simulink model "test_newfft_4"  (Simulink 7.0)
settings: Solver=ode45  StartTime=0.0  StopTime=100  RelTol=1e-3
libraries: xbsIndex_r4 x135, simulink x1, casper_library x1
(part 1 of 3)
settings Model: Creator=homin  LastModifiedBy=homin
settings DebuggingCC: SaveWithParameterizedLinksMsg=none  SignalResolutionControl=TryResolveAllWithWarning  MultiTaskDSMMsg=warning  MultiTaskCondExecSysMsg=none  StrictBusMsg=None
settings RTWCC: IncludeERTFirstTime=on
settings GRTTargetCC: TargetFcnLib=ansi_tfl_tmw.mat

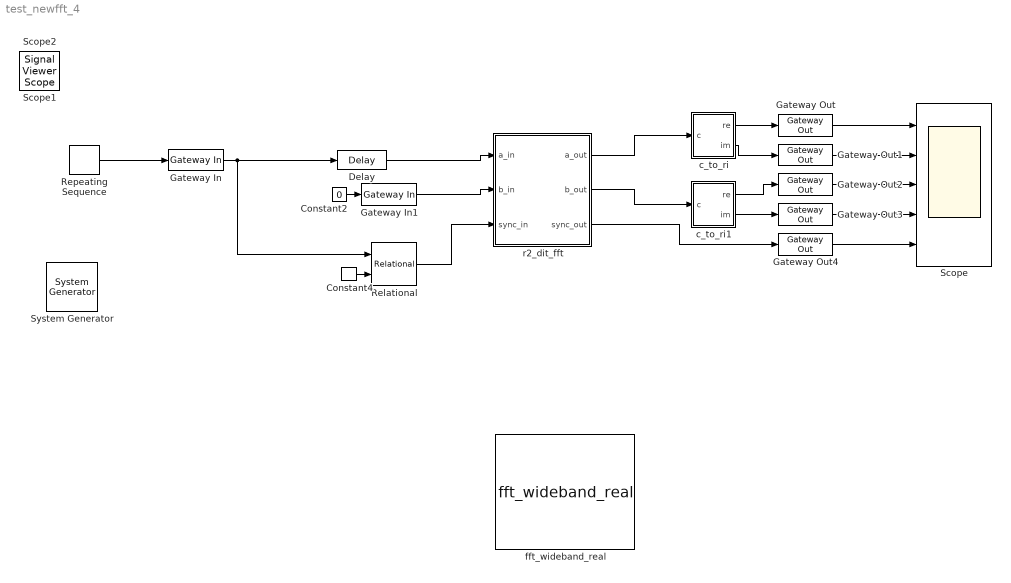
== system test_newfft_4 ==
  " System Generator" : xbsIndex_r4/ System Generator  Tag=genX  SystemSampleTime=-1  xilinxfamily=Virtex2  part=xc2v1000  speed=-4  package=bg575  synthesis_tool=XST  clock_wrapper=Clock Enables  directory=./netlist  testbench=off  simulink_period=1  sysclk_period=100  dcm_input_clock_period=100  incr_netlist=off  trim_vbits=Everywhere in SubSystem  dbl_ovrd=According to Block Masks  core_generation=According to Block Masks  run_coregen=off  deprecated_control=off  eval_field=0  block_type=sysgen
      settings: block_version=10.1.3
  Constant2 : Constant  Value=0  OutDataType=sfix(16)  OutScaling=2^0
  Constant4 : xbsIndex_r4/Constant  arith_type=Unsigned  const=0  n_bits=16  bin_pt=0  explicit_period=off  period=1  equ=P=C  opselect=C  inp2=PCIN>>17  opr=+  inp1=P  carry=CIN  dbl_ovrd=off  block_type=constant
  Delay : xbsIndex_r4/Delay  en=off  latency=2  dbl_ovrd=off  reg_retiming=off  block_type=delay
      settings: xl_area=[0, 0, 0, 0, 0, 0, 0]
  Gateway In : xbsIndex_r4/Gateway In  arith_type=Unsigned  n_bits=16  bin_pt=0  quantization=Truncate  overflow=Wrap  period=1  dbl_ovrd=off  timing_constraint=None  locs_specified=off  LOCs={}  block_type=gatewayin
      settings: infoedit="Gateway in block.  Converts inputs of type Simulink integer, double and fixed point to  Xilinx fixed point type.<P><P>Hardware notes:  In hardware these blocks become top level input ports."  xl_area=[0, 0, 0, 0, 0, 0, 0]  block_version=10.1.3
  Gateway In1 : xbsIndex_r4/Gateway In  arith_type=Unsigned  n_bits=16  bin_pt=0  quantization=Truncate  overflow=Wrap  period=1  dbl_ovrd=off  timing_constraint=None  locs_specified=off  LOCs={}  block_type=gatewayin
      settings: infoedit="Gateway in block.  Converts inputs of type Simulink integer, double and fixed point to  Xilinx fixed point type.<P><P>Hardware notes:  In hardware these blocks become top level input ports."  xl_area=[0, 0, 0, 0, 0, 0, 0]  block_version=10.1.3
  Gateway Out{,1..4} (5 alike) : xbsIndex_r4/Gateway Out  hdl_port=on  timing_constraint=None  locs_specified=off  LOCs={}  block_type=gatewayout
      settings: infoedit="Gateway out block.  Converts Xilinx fixed point inputs into ouputs of type Simulink integer, double, or fixed point.<P><P>Hardware notes:  In hardware these blocks become top level output ports or are discarded, depending on how they are configured."  xl_area=[0, 0, 0, 0, 0, 0, 0]  block_version=10.1.3
  Relational : xbsIndex_r4/Relational  mode=a!=b  en=off  latency=0  dbl_ovrd=off  block_type=relational
      settings: xl_area=[0, 0, 0, 0, 0, 0, 0]  block_version=10.1.3
  Repeating Sequence : simulink/Sources/Repeating Sequence  SystemSampleTime=-1  rep_seq_t=[0:16]  rep_seq_y=[1 zeros(1,15) 1]*hex2dec('7f00')
  Scope : Scope  NumInputPorts=5
      settings: YMin=-5~-5~-5~-5~-5  YMax=5~5~5~5~5
  c_to_ri : Subsystem  mask(Complex to Real-Imag){n_bits=10, bin_pt=7}
      mask prompts: n_bits "Bit Width"; bin_pt "Binary Point"
      mask help: Outputs real and imaginary components of a complex input.
      mask init:
      | c_to_ri_init(gcb,n_bits,bin_pt);
      settings: AttributesFormatString=10_7 r/i
      mask Help:
      | <pre>
      | Description::
      | 
      | Outputs real and imaginary components of a complex input.
      | Useful for simplifying interconnects.
      | See also: Real-Imag to Complex (ri_to_c)
      | 
      | Mask Parameters::
      | 
      | Bit Width (n_bits): Specifies the width of the real/imaginary components.
      | Assumed equal for both components.
      | 
      | Binary Point (bin_pt): Specifies the binary point location in the real/imaginary components.
      | Assumed equal for both components.
      | </pre>
  c_to_ri1 : Subsystem  mask(Complex to Real-Imag){n_bits=10, bin_pt=7}
      mask prompts: n_bits "Bit Width"; bin_pt "Binary Point"
      mask help: Outputs real and imaginary components of a complex input.
      mask init:
      | c_to_ri_init(gcb,n_bits,bin_pt);
      settings: AttributesFormatString=10_7 r/i
      mask Help:
      | <pre>
      | Description::
      | 
      | Outputs real and imaginary components of a complex input.
      | Useful for simplifying interconnects.
      | See also: Real-Imag to Complex (ri_to_c)
      | 
      | Mask Parameters::
      | 
      | Bit Width (n_bits): Specifies the width of the real/imaginary components.
      | Assumed equal for both components.
      | 
      | Binary Point (bin_pt): Specifies the binary point location in the real/imaginary components.
      | Assumed equal for both components.
      | </pre>
  fft_wideband_real : casper_library/FFTs/fft_wideband_real  SystemSampleTime=-1  FFTSize=5  input_bit_width=18  coeff_bit_width=18  n_inputs=2  quantization=Truncate  overflow=Wrap  add_latency=2  mult_latency=3  bram_latency=2  arch=Virtex2Pro  opt_target=Multipliers  coeffs_bit_limit=8  delays_bit_limit=9  specify_mult=off  mult_spec=[2 2 2 2 2]  dsp48_adders=off
      link override fft_direct/butterfly1_0/convert_of1/all_0s: logical_function=NAND  inputs=5  latency=latency  precision=Full
      link override fft_direct/butterfly1_0/convert_of1/all_1s: logical_function=NAND  inputs=5  latency=latency  precision=Full
      link override fft_direct/butterfly1_0/convert_of1/and: logical_function=AND  inputs=2  latency=0  precision=Full
      link override fft_direct/butterfly1_0/convert_of1/convert: n_bits=bit_width_o  bin_pt=binary_point_o  quantization=Truncate  overflow=Wrap  latency=latency  pipeline=on
      link override fft_direct/butterfly1_0/convert_of1/din: Port=1
      link override fft_direct/butterfly1_0/convert_of1/dout: Port=1
      link override fft_direct/butterfly1_0/convert_of1/of: Port=2
      link override fft_direct/butterfly1_0/convert_of1/slice1: boolean_output=on  mode=Upper Bit Location + Width  bit1=0  base1=MSB of Input
      link override fft_direct/butterfly1_0/convert_of1/slice2: boolean_output=on  mode=Upper Bit Location + Width  bit1=-1  base1=MSB of Input
      link override fft_direct/butterfly1_0/convert_of1/slice3: boolean_output=on  mode=Upper Bit Location + Width  bit1=-2  base1=MSB of Input
      link override fft_direct/butterfly1_0/convert_of1/slice4: boolean_output=on  mode=Upper Bit Location + Width  bit1=-3  base1=MSB of Input
      link override fft_direct/butterfly1_0/convert_of1/slice5: boolean_output=on  mode=Upper Bit Location + Width  bit1=-4  base1=MSB of Input
      link override fft_direct/butterfly1_0/convert_of2/all_0s: logical_function=NAND  inputs=5  latency=latency  precision=Full
      link override fft_direct/butterfly1_0/convert_of2/all_1s: logical_function=NAND  inputs=5  latency=latency  precision=Full
      link override fft_direct/butterfly1_0/convert_of2/and: logical_function=AND  inputs=2  latency=0  precision=Full
      link override fft_direct/butterfly1_0/convert_of2/convert: n_bits=bit_width_o  bin_pt=binary_point_o  quantization=Truncate  overflow=Wrap  latency=latency  pipeline=on
      link override fft_direct/butterfly1_0/convert_of2/din: Port=1
      link override fft_direct/butterfly1_0/convert_of2/dout: Port=1
      link override fft_direct/butterfly1_0/convert_of2/of: Port=2
      link override fft_direct/butterfly1_0/convert_of2/slice1: boolean_output=on  mode=Upper Bit Location + Width  bit1=0  base1=MSB of Input
      link override fft_direct/butterfly1_0/convert_of2/slice2: boolean_output=on  mode=Upper Bit Location + Width  bit1=-1  base1=MSB of Input
      link override fft_direct/butterfly1_0/convert_of2/slice3: boolean_output=on  mode=Upper Bit Location + Width  bit1=-2  base1=MSB of Input
      link override fft_direct/butterfly1_0/convert_of2/slice4: boolean_output=on  mode=Upper Bit Location + Width  bit1=-3  base1=MSB of Input
      link override fft_direct/butterfly1_0/convert_of2/slice5: boolean_output=on  mode=Upper Bit Location + Width  bit1=-4  base1=MSB of Input
      link override fft_direct/butterfly1_0/convert_of3/all_0s: logical_function=NAND  inputs=5  latency=latency  precision=Full
      link override fft_direct/butterfly1_0/convert_of3/all_1s: logical_function=NAND  inputs=5  latency=latency  precision=Full
      link override fft_direct/butterfly1_0/convert_of3/and: logical_function=AND  inputs=2  latency=0  precision=Full
      link override fft_direct/butterfly1_0/convert_of3/convert: n_bits=bit_width_o  bin_pt=binary_point_o  quantization=Truncate  overflow=Wrap  latency=latency  pipeline=on
      link override fft_direct/butterfly1_0/convert_of3/din: Port=1
      link override fft_direct/butterfly1_0/convert_of3/dout: Port=1
      link override fft_direct/butterfly1_0/convert_of3/of: Port=2
      link override fft_direct/butterfly1_0/convert_of3/slice1: boolean_output=on  mode=Upper Bit Location + Width  bit1=0  base1=MSB of Input
      link override fft_direct/butterfly1_0/convert_of3/slice2: boolean_output=on  mode=Upper Bit Location + Width  bit1=-1  base1=MSB of Input
      link override fft_direct/butterfly1_0/convert_of3/slice3: boolean_output=on  mode=Upper Bit Location + Width  bit1=-2  base1=MSB of Input
      link override fft_direct/butterfly1_0/convert_of3/slice4: boolean_output=on  mode=Upper Bit Location + Width  bit1=-3  base1=MSB of Input
      link override fft_direct/butterfly1_0/convert_of3/slice5: boolean_output=on  mode=Upper Bit Location + Width  bit1=-4  base1=MSB of Input
      link override fft_direct/butterfly1_0/convert_of4/all_0s: logical_function=NAND  inputs=5  latency=latency  precision=Full
      link override fft_direct/butterfly1_0/convert_of4/all_1s: logical_function=NAND  inputs=5  latency=latency  precision=Full
      link override fft_direct/butterfly1_0/convert_of4/and: logical_function=AND  inputs=2  latency=0  precision=Full
      link override fft_direct/butterfly1_0/convert_of4/convert: n_bits=bit_width_o  bin_pt=binary_point_o  quantization=Truncate  overflow=Wrap  latency=latency  pipeline=on
      link override fft_direct/butterfly1_0/convert_of4/din: Port=1
      link override fft_direct/butterfly1_0/convert_of4/dout: Port=1
      link override fft_direct/butterfly1_0/convert_of4/of: Port=2
      link override fft_direct/butterfly1_0/convert_of4/slice1: boolean_output=on  mode=Upper Bit Location + Width  bit1=0  base1=MSB of Input
      link override fft_direct/butterfly1_0/convert_of4/slice2: boolean_output=on  mode=Upper Bit Location + Width  bit1=-1  base1=MSB of Input
      link override fft_direct/butterfly1_0/convert_of4/slice3: boolean_output=on  mode=Upper Bit Location + Width  bit1=-2  base1=MSB of Input
      link override fft_direct/butterfly1_0/convert_of4/slice4: boolean_output=on  mode=Upper Bit Location + Width  bit1=-3  base1=MSB of Input
      link override fft_direct/butterfly1_0/convert_of4/slice5: boolean_output=on  mode=Upper Bit Location + Width  bit1=-4  base1=MSB of Input
      link override fft_direct/butterfly1_0/twiddle/convert_of/convert: n_bits=bit_width_o  bin_pt=binary_point_o  quantization=Truncate  overflow=Wrap  latency=latency  pipeline=on
      link override fft_direct/butterfly1_0/twiddle/convert_of/din: Port=1
      link override fft_direct/butterfly1_0/twiddle/convert_of/dout: Port=1
      link override fft_direct/butterfly1_0/twiddle/convert_of/never: arith_type=Boolean  const=0  explicit_period=on  period=1
      link override fft_direct/butterfly1_0/twiddle/convert_of/of: Port=2
      link override fft_direct/butterfly1_0/twiddle/convert_of1/convert: n_bits=bit_width_o  bin_pt=binary_point_o  quantization=Truncate  overflow=Wrap  latency=latency  pipeline=on
      link override fft_direct/butterfly1_0/twiddle/convert_of1/din: Port=1
      link override fft_direct/butterfly1_0/twiddle/convert_of1/dout: Port=1
      link override fft_direct/butterfly1_0/twiddle/convert_of1/never: arith_type=Boolean  const=0  explicit_period=on  period=1
      link override fft_direct/butterfly1_0/twiddle/convert_of1/of: Port=2
      link override fft_direct/butterfly1_0/twiddle/convert_of2/convert: n_bits=bit_width_o  bin_pt=binary_point_o  quantization=Truncate  overflow=Wrap  latency=latency  pipeline=on
      link override fft_direct/butterfly1_0/twiddle/convert_of2/din: Port=1
      link override fft_direct/butterfly1_0/twiddle/convert_of2/dout: Port=1
      link override fft_direct/butterfly1_0/twiddle/convert_of2/never: arith_type=Boolean  const=0  explicit_period=on  period=1
      link override fft_direct/butterfly1_0/twiddle/convert_of2/of: Port=2
      settings: AttributesFormatString=FFTSize=5
  r2_dit_fft : Subsystem  AncestorBlock=newfft_library/FFT/r2_dit_fft  mask(Biplex Radix-2 DIT FFT){n_stages=2, n_bits=8, bin_pt=7, shifts=[0], commutator_bram=0, twiddle_bram=0, n_bits_w=9, mult_latency=3, add_latency=1, commute_output=Yes (SLR16), output_order=Normal, show_sbo=on, munge_submasks=DumbDown}
      mask prompts: n_stages "Total Stages"; n_bits "Number of Bits In"; bin_pt "Binary Point In"; shifts "Shifting Schedule"; commutator_bram "Number of Stages Using BRAM for Biplex Commutators (i.e. delays)"; twiddle_bram "Number of Stages Using BRAM for Twiddle Coefficients"; n_bits_w "Twiddle Coefficient Bitwidth"; mult_latency "Multiplier Latency"; add_latency "Adder Latency"; commute_output "Commute Output"; output_order "Output Order"; show_sbo "Show Sub-Block Options"; munge_submasks "Sub-Block Masks"
      mask help: A biplex radix-2 decimation-in-time Fast Fourier Transform.
      mask init:
      | tic
      | r2_dit_fft_init(gcb, ...
      |   n_stages, ...
      |   n_bits, ...
      |   bin_pt, ...
      |   shifts, ...
      |   commutator_bram, ...
      |   twiddle_bram, ...
      |   n_bits_w, ...
      |   mult_latency, ...
      |   add_latency, ...
      |   commute_output, ...
      |   output_order, ...
      |   lower(get_param(gcb,'munge_submasks')) );
      | disp('r2_dit_fft initialization complete.');
      | toc
      settings: AttributesFormatString=|
      | 4 points
      | 8_7 r/i in
      | 9_7 twiddles
      mask Help:
      | <pre>
      | Description::
      | 
      | A biplex radix-2 decimation-in-time Fast Fourier Transform.
      | 
      | The two inputs to the biplex FFT are independent complex signals (e.g. A and B).
      | 
      | Without an output commutator, the two outputs of the FFT are commuted such that the a_out
      | signal is really the "lower" half of A's transform followed by the "lower" half of B's
      | transform and b_out is really the "upper" half of A's transform followed by the "upper"
      | half of B's transform.
      | 
      | If it is desired to have the two halves of A's transform follow each other on the same path
      | and the two halves of B's transform follow each other on the same path, then be sure to
      | check the "Output Commutator" checkbox.  This will result in the "lower" half of A (or B)
      | followed by the "upper" half of A (or B).  Including the output commutator uses additional
      | resources.
      | 
      | If the "Normal" Ouput Order option is chosen, the output will be in normal order (though still in
      | commuted halves if no output commutator is used).  If the "Bit Reversed" Output Order" option is
      | selected, the output halves (either commuted or not) will each be in bit reversed order
      | (i.e. each half of each transform will be in bit reversed output order).   Normal output is easier
      | for humans to work with (especially for testing), but it uses additional resources.  Bit reversed
      | output is the implementation's inhernet output order so that option uses no additional resources.
      | 
      | The number of bits for each real and imaginary component grows by two through each stage.
      | If a stage's input bit width is 17 or less, three embedded multipliers will be used per complex multiply.
      | If a stage's input bit width is 18, four embedded multipliers will be used per complex multiply.
      | If a stage's input bit width exceeds 18, then substantially more embedded multipliers will be used
      | per complex multiply.  Enabling "shifting" in some (or all) stages can limit the bit growth
      | to prevent this.  See the Shifting Schedule parameter for more info.
      | 
      | Mask Parameters::
      | 
      | Total Stages (n_stages):  The number of total stages in the FFT.
      | The FFT will have 2^n_stages points.
      | 
      | Number of Bits In (n_bits): Specifies the width of the real/imaginary components of ports
      | a_in and b_in.  Assumed equal for both components.  The output bit width will be
      | n_bits+n_stages (assuming sum(shifts)==0).
      | 
      | Binary Point In (bin_pt): Specifies the binary point position of the real/imaginary
      | components of ports a_in and b_in.  Assumed equal for both components.
      | 
      | Shifting Schedule (shifts): A vector specifying how many bits to shift by at each stage.
      | Missing values are assumed to be zero; extra values are ignored.
      | 
      | Number of Stages Using BRAM for Biplex Commutators (commutator_bram): Number of stages
      | that will use BRAM for commutator memory.  Remaining stages will use SLR16 elements (slices).
      | 
      | Number of Stages Using BRAM for Twiddle Coefficients (twiddle_bram): Number of stages that
      | will use BRAM for twiddle coeeficient storage.  Remaining stages will use distributed memory
      | (slices).
      | 
      | Twiddle Coefficient Bitwidth (n_bits_w): Specifies the width of the real/imaginary
      | components of the twiddle coefficients.  Assumed equal for both components.
      | 
      | Multiplier Latency (mult_latency): Latency to use for the underlying real multipliers.
      | 
      | Adder Latency (add_latency): Latency to use for the underlying real adders.
      | 
      | Commute Output (commute_output): Popup options for an output commutator.  See decription
      | above for details on the output commutator.  Choices are:
      |     "No" - No output commutator
      |     "Yes (SLR16)" - Include output commutator using SLR16 elements
      |     "Yes (BRAM)" - Include output commutator using BRAM
      | 
      | Output Order (output_order): Popup options for selecting the output order.  See description
      | above for details on the output order.  Choices are:
      |     "Bit Reversed" - Output each half of each transform in bit reversed order.
      |     "Normal" - Output each half of each transform in normal order.
      | </pre>
      mask StyleString: edit,edit,edit,edit,edit,edit,edit,edit,edit,popup(No|Yes (SLR16)|Yes (BRAM)),popup(Bit Reversed|Normal),checkbox,popup(Keep|DumbDown|Unmask)
      mask CallbackString:
      | |||||||||||mvs=get_param(gcb,'MaskVisibilityString');
      | if strcmp(get_param(gcb,'show_sbo'),'on')
      |   onoff='on';
      | else
      |   onoff='off';
      | end
      | mvs=regexprep(mvs,'o[nf]*$',onoff);
      | set_param(gcb,'MaskVisibilityString',mvs);
      | |mvs=get_param(gcb,'MaskVisibilityString');
      | if strcmp(get_param(gcb,'show_sbo'),'on')
      |   onoff='on';
      | else
      |   onoff='off';
      | end
      | mvs=regexprep(mvs,'o[nf]*$',onoff);
      | set_param(gcb,'MaskVisibilityString',mvs);
  Scope1 : SignalViewerScope  IOType=viewer  NumInputPorts=5  RefreshTime=0.035000
      settings: YMin=-5~-5~-5~-5~-5  YMax=5~5~5~5~5
  Scope2 : SignalViewerScope  IOType=viewer  NumInputPorts=5  RefreshTime=0.035000
      settings: ShowLegends=on  YMin=-5~-5~-5~-5~-5  YMax=5~5~5~5~5
  wires:
  Gateway In/1 -> Relational/1, Delay/1
  Gateway In1/1 -> r2_dit_fft/2(b_in)
  Relational/1 -> r2_dit_fft/3(sync_in)
  Constant2/1 -> Gateway In1/1
  Gateway Out/1 -> Scope/1
  Gateway Out1/1 -> Scope/2
  Gateway Out2/1 -> Scope/3
  Constant4/1 -> Relational/2
  Repeating Sequence/1 -> Gateway In/1
  Delay/1 -> r2_dit_fft/1(a_in)
  Gateway Out3/1 -> Scope/4
  Gateway Out4/1 -> Scope/5
  c_to_ri/1(re) -> Gateway Out/1
  c_to_ri/2(im) -> Gateway Out1/1
  c_to_ri1/1(re) -> Gateway Out2/1
  c_to_ri1/2(im) -> Gateway Out3/1
  r2_dit_fft/1(a_out) -> c_to_ri/1(c)
  r2_dit_fft/2(b_out) -> c_to_ri1/1(c)
  r2_dit_fft/3(sync_out) -> Gateway Out4/1

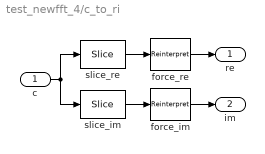
== system test_newfft_4/c_to_ri ==
  c : Inport  OutDataType=sfix(16)  OutScaling=2^0
  force_im : xbsIndex_r4/Reinterpret  force_arith_type=on  arith_type="Signed  (2's comp)"  force_bin_pt=on  bin_pt=7  block_type=reinterpret
      settings: infoedit="Changes signal type without altering the binary representation.   You can changed the signal between signed and unsigned, and relocate the binary point.<P><P>Hardware notes: In hardware this block costs nothing.<P><P>Example:  Suppose the input is 6 bits wide, signed, with 2 fractional bits, and the output is forced to unsigned with 0 fractional bits.  Then an input of -2.0 (1110.00 in binary 2's complement) becomes an output of 56 (111000 in binary)."  block_version=10.1.3
  force_re : xbsIndex_r4/Reinterpret  force_arith_type=on  arith_type="Signed  (2's comp)"  force_bin_pt=on  bin_pt=7  block_type=reinterpret
      settings: infoedit="Changes signal type without altering the binary representation.   You can changed the signal between signed and unsigned, and relocate the binary point.<P><P>Hardware notes: In hardware this block costs nothing.<P><P>Example:  Suppose the input is 6 bits wide, signed, with 2 fractional bits, and the output is forced to unsigned with 0 fractional bits.  Then an input of -2.0 (1110.00 in binary 2's complement) becomes an output of 56 (111000 in binary)."  block_version=10.1.3
  slice_im : xbsIndex_r4/Slice  nbits=10  boolean_output=off  mode=Lower Bit Location + Width  bit1=0  base1=MSB of Input  bit0=0  base0=LSB of Input  dbl_ovrd=off  block_type=slice
      settings: infoedit="Extracts a given range of bits from each input sample and presents it at the output.  The output type is ordinarily unsigned with binary point at zero, but can be Boolean when the slice is one bit wide.<P><P>Hardware notes: In hardware this block costs nothing."  block_version=10.1.3
  slice_re : xbsIndex_r4/Slice  nbits=10  boolean_output=off  mode=Upper Bit Location + Width  bit1=0  base1=MSB of Input  bit0=0  base0=LSB of Input  dbl_ovrd=off  block_type=slice
      settings: infoedit="Extracts a given range of bits from each input sample and presents it at the output.  The output type is ordinarily unsigned with binary point at zero, but can be Boolean when the slice is one bit wide.<P><P>Hardware notes: In hardware this block costs nothing."  block_version=10.1.3
  re : Outport  OutDataType=sfix(16)  OutScaling=2^0
  im : Outport  Port=2  OutDataType=sfix(16)  OutScaling=2^0
  wires:
  slice_re/1 -> force_re/1
  slice_im/1 -> force_im/1
  force_re/1 -> re/1
  force_im/1 -> im/1
  c/1 -> slice_re/1, slice_im/1

== system test_newfft_4/c_to_ri1 ==
  c : Inport  OutDataType=sfix(16)  OutScaling=2^0
  force_im : xbsIndex_r4/Reinterpret  force_arith_type=on  arith_type="Signed  (2's comp)"  force_bin_pt=on  bin_pt=7  block_type=reinterpret
      settings: infoedit="Changes signal type without altering the binary representation.   You can changed the signal between signed and unsigned, and relocate the binary point.<P><P>Hardware notes: In hardware this block costs nothing.<P><P>Example:  Suppose the input is 6 bits wide, signed, with 2 fractional bits, and the output is forced to unsigned with 0 fractional bits.  Then an input of -2.0 (1110.00 in binary 2's complement) becomes an output of 56 (111000 in binary)."  block_version=10.1.3
  force_re : xbsIndex_r4/Reinterpret  force_arith_type=on  arith_type="Signed  (2's comp)"  force_bin_pt=on  bin_pt=7  block_type=reinterpret
      settings: infoedit="Changes signal type without altering the binary representation.   You can changed the signal between signed and unsigned, and relocate the binary point.<P><P>Hardware notes: In hardware this block costs nothing.<P><P>Example:  Suppose the input is 6 bits wide, signed, with 2 fractional bits, and the output is forced to unsigned with 0 fractional bits.  Then an input of -2.0 (1110.00 in binary 2's complement) becomes an output of 56 (111000 in binary)."  block_version=10.1.3
  slice_im : xbsIndex_r4/Slice  nbits=10  boolean_output=off  mode=Lower Bit Location + Width  bit1=0  base1=MSB of Input  bit0=0  base0=LSB of Input  dbl_ovrd=off  block_type=slice
      settings: infoedit="Extracts a given range of bits from each input sample and presents it at the output.  The output type is ordinarily unsigned with binary point at zero, but can be Boolean when the slice is one bit wide.<P><P>Hardware notes: In hardware this block costs nothing."  block_version=10.1.3
  slice_re : xbsIndex_r4/Slice  nbits=10  boolean_output=off  mode=Upper Bit Location + Width  bit1=0  base1=MSB of Input  bit0=0  base0=LSB of Input  dbl_ovrd=off  block_type=slice
      settings: infoedit="Extracts a given range of bits from each input sample and presents it at the output.  The output type is ordinarily unsigned with binary point at zero, but can be Boolean when the slice is one bit wide.<P><P>Hardware notes: In hardware this block costs nothing."  block_version=10.1.3
  re : Outport  OutDataType=sfix(16)  OutScaling=2^0
  im : Outport  Port=2  OutDataType=sfix(16)  OutScaling=2^0
  wires:
  slice_re/1 -> force_re/1
  slice_im/1 -> force_im/1
  force_re/1 -> re/1
  force_im/1 -> im/1
  c/1 -> slice_re/1, slice_im/1

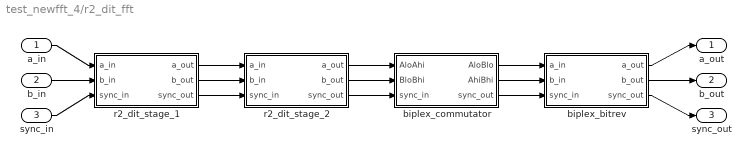
== system test_newfft_4/r2_dit_fft ==
  a_in : Inport  OutDataType=sfix(16)  OutScaling=2^0
  b_in : Inport  Port=2  OutDataType=sfix(16)  OutScaling=2^0
  sync_in : Inport  Port=3  OutDataType=sfix(16)  OutScaling=2^0
  biplex_bitrev : Subsystem  mask(Biplex Bit Reverse Reorder){log2_size=1, n_bits=10}
      mask prompts: log2_size "Log2 Block Size"; n_bits "Number of Bits"
      mask help: Reorders the input sequence from normal order to bit reverse order (or vise versa).
      settings: AttributesFormatString=size = 2
      mask Help:
      | <pre>
      | Description::
      | 
      | Reorders the input sequence from normal order to bit reverse order (or vise versa).
      | 
      | Mask Parameters::
      | 
      | Log 2 Block Size (log2_size): The base-2 logarithm of the length of one complete input block.
      | This MUST be an integer because the current implementation requires that
      | the input block size MUST be a power of 2.  (aka "N")
      | 
      | Number of Bits (n_bits): Specifies the width of the real/imaginary components.
      | Width of each component is assumed equal.
      | </pre>
  biplex_commutator : Subsystem  mask(Biplex Commutator){log2_size=2, n_bits=10, use_bram=off}
      mask prompts: log2_size "Log2 Block Size"; n_bits "Bit Width"; use_bram "Use BRAM"
      mask help: The biplex commutator commutes the first half of the BloBhi input "block" with the last half of the AloAhi input "block". A "block" is 2^log2_size consecutive samples (i.e. always a power of 2). sync_in precedes the first data input sample by one clock cycle. Overall latency from sync_in to sync_out is 2^(log2_size-1)+1.
      settings: AttributesFormatString=|
      | size = 4
      | delay slr
      mask Help:
      | <pre>
      | Description::
      | 
      | The biplex commutator commutes the first half of the BloBhi input "block"  with the last half
      | of the AloAhi input "block".  A "block" is 2^log2_size consecutive samples (i.e. always a
      | power of 2).
      | 
      | sync_in precedes the first data input sample by one clock cycle.
      | sync_out precedes the corresponding output sample by one clock cycle.
      | Overall latency from sync_in to sync_out is 2^(N-1)+1.
      | 
      | Mask Parameters::
      | 
      | Log 2 Block Size (log2_size): The base-2 logarithm of the length of one complete input block.
      | This MUST be an integer because the current implementation requires that
      | the input block size MUST be a power of 2.  (aka "N")
      | 
      | Bit Width (n_bits): Specifies the width of the real/imaginary components.
      | Width of each component is assumed equal.
      | 
      | Use BRAM (use_bram): Check this checkbox to implement the internal delays using BRAM.
      | If unchecked, the internal delays will be implemented using SLR16 elements.
      | </pre>
  r2_dit_stage_1 : Subsystem  mask(Radix-2 DIT FFT Stage){n_stages=2, cur_stage=1, n_bits=8, bin_pt=7, shift=0, commutator_bram=off, twiddle_bram=off, n_bits_w=9, mult_latency=3, add_latency=1}
      mask prompts: n_stages "Total Stages (2^N points)"; cur_stage "Current Stage"; n_bits "Number of Bits In"; bin_pt "Binary Point In"; shift "Shift Bits"; commutator_bram "Use BRAM for Biplex Commutator"; twiddle_bram "Use BRAM For Twiddle Coefficients"; n_bits_w "Twiddle Coefficient Bitwidth"; mult_latency "Multiplier Latency"; add_latency "Adder Latency"
      mask help: A radix-2 decimation-in-time Fast Fourier Transform stage.
      settings: AttributesFormatString=|
      | stage 1 of 2
      | delay slr
      | twiddle dist
      | shift 0
      mask Help:
      | <pre>
      | Description::
      | 
      | A radix-2 decimation-in-time Fast Fourier Transform stage.
      | 
      | This radix-2 decimation-in-time FFT stage is designed to be daisy chained together
      | to form a multi-stage FFT.  The resulting FFT will have (2^n_stages) points.
      | 
      | The two inputs to the chain are independent complex signals (e.g. A and B).
      | 
      | The two outputs of the last stage of the chain are commuted such that the a_out signal is really
      | the "lower" half of A's transform followed by the "lower" half of B's transform and b_out is really
      | the "upper" half of A's transform followed by the "upper" half of B's transform.  Each half is in bit-reversed order.
      | 
      | If it is desired to have the two halves of A's transform follow each other on the same path and
      | the two halves of B's transform follow each other on the same path, then a_out and b_out can
      | be fed through a biplex_commutator with block size 2^n_stages.  This will result in the "lower"
      | half of A (or B) followed by the "upper" half of A (or B), but note that each half of A (or B)
      | will still remain in bit-reversed order (i.e. each output is bit-reversed in halves; it is not bit reversed
      | in its entirety).
      | 
      | The number of bits for each real and imaginary component grows by one through this stage.
      | If the input bit width is 17 or less, three embedded multipliers will be used per complex multiply.
      | If the input bit width is 18, four embedded multipliers will be used per complex multiply.
      | If the input bit width exceeds 18, then substantially more embedded multipliers will be used
      | per complex multiply.  Enabling "shifting" in some (or all) stages can limit the bit growth
      | to prevent this.
      | 
      | Mask Parameters::
      | 
      | Total Stages (n_stages):  The number of total stages in the FFT.
      | The FFT will have 2^n_stages points.
      | 
      | Current Stage (cur_stage):  The number of the current stage.  Note that stages are counted
      | from 1 to n_stages for DIT (i.e. cur_stage==1 for the first stage).
      | 
      | Number of Bits In (n_bits): Specifies the width of the real/imaginary components of ports
      | a_in and b_in.  Assumed equal for both components.  The real/imaginary components of
      | oorts a_out and b_out will be one bit wider.
      | 
      | Binary Point In (bin_pt): Specifies the binary point position of the real/imaginary
      | components of ports a_in and b_in.  Assumed equal for both components.
      | 
      | Shift Bits (shift): Specifies how many bits to shift (down) by.  A positive value causes
      | the specified number of least significant bits to be dropped.  Usually zero or positive values
      | are used to permit or limit bit growth, but negative values can be used to induce bit growth.
      | 
      | Use BRAM for Biplex Commutator (commutator_bram): Check this checkbox to implement
      | the biplex commutator using BRAM.  If unchecked, the biplex commutator will be implemented
      | using SLR16 elements (i.e. slices).
      | 
      | Use BRAM for Twiddle Coefficients (twiddle_bram): Check this checkbox to store twiddle
      | coefficients in BRAM.  If unchecked, the twiddle coefficients will be sored in distributed
      | memory (i.e. slices).
      | 
      | Twiddle Coefficient Bitwidth (n_bits_w): Specifies the width of the real/imaginary
      | components of the twiddle coefficients.  Assumed equal for both components.
      | 
      | Multiplier Latency (mult_latency): Latency to use for the underlying real multipliers.
      | 
      | Adder Latency (add_latency): Latency to use for the underlying real adders.
      | </pre>
  r2_dit_stage_2 : Subsystem  mask(Radix-2 DIT FFT Stage){n_stages=2, cur_stage=2, n_bits=9, bin_pt=7, shift=0, commutator_bram=off, twiddle_bram=off, n_bits_w=9, mult_latency=3, add_latency=1}
      mask prompts: n_stages "Total Stages (2^N points)"; cur_stage "Current Stage"; n_bits "Number of Bits In"; bin_pt "Binary Point In"; shift "Shift Bits"; commutator_bram "Use BRAM for Biplex Commutator"; twiddle_bram "Use BRAM For Twiddle Coefficients"; n_bits_w "Twiddle Coefficient Bitwidth"; mult_latency "Multiplier Latency"; add_latency "Adder Latency"
      mask help: A radix-2 decimation-in-time Fast Fourier Transform stage.
      settings: AttributesFormatString=|
      | stage 2 of 2
      | delay slr
      | twiddle dist
      | shift 0
      mask Help:
      | <pre>
      | Description::
      | 
      | A radix-2 decimation-in-time Fast Fourier Transform stage.
      | 
      | This radix-2 decimation-in-time FFT stage is designed to be daisy chained together
      | to form a multi-stage FFT.  The resulting FFT will have (2^n_stages) points.
      | 
      | The two inputs to the chain are independent complex signals (e.g. A and B).
      | 
      | The two outputs of the last stage of the chain are commuted such that the a_out signal is really
      | the "lower" half of A's transform followed by the "lower" half of B's transform and b_out is really
      | the "upper" half of A's transform followed by the "upper" half of B's transform.  Each half is in bit-reversed order.
      | 
      | If it is desired to have the two halves of A's transform follow each other on the same path and
      | the two halves of B's transform follow each other on the same path, then a_out and b_out can
      | be fed through a biplex_commutator with block size 2^n_stages.  This will result in the "lower"
      | half of A (or B) followed by the "upper" half of A (or B), but note that each half of A (or B)
      | will still remain in bit-reversed order (i.e. each output is bit-reversed in halves; it is not bit reversed
      | in its entirety).
      | 
      | The number of bits for each real and imaginary component grows by one through this stage.
      | If the input bit width is 17 or less, three embedded multipliers will be used per complex multiply.
      | If the input bit width is 18, four embedded multipliers will be used per complex multiply.
      | If the input bit width exceeds 18, then substantially more embedded multipliers will be used
      | per complex multiply.  Enabling "shifting" in some (or all) stages can limit the bit growth
      | to prevent this.
      | 
      | Mask Parameters::
      | 
      | Total Stages (n_stages):  The number of total stages in the FFT.
      | The FFT will have 2^n_stages points.
      | 
      | Current Stage (cur_stage):  The number of the current stage.  Note that stages are counted
      | from 1 to n_stages for DIT (i.e. cur_stage==1 for the first stage).
      | 
      | Number of Bits In (n_bits): Specifies the width of the real/imaginary components of ports
      | a_in and b_in.  Assumed equal for both components.  The real/imaginary components of
      | oorts a_out and b_out will be one bit wider.
      | 
      | Binary Point In (bin_pt): Specifies the binary point position of the real/imaginary
      | components of ports a_in and b_in.  Assumed equal for both components.
      | 
      | Shift Bits (shift): Specifies how many bits to shift (down) by.  A positive value causes
      | the specified number of least significant bits to be dropped.  Usually zero or positive values
      | are used to permit or limit bit growth, but negative values can be used to induce bit growth.
      | 
      | Use BRAM for Biplex Commutator (commutator_bram): Check this checkbox to implement
      | the biplex commutator using BRAM.  If unchecked, the biplex commutator will be implemented
      | using SLR16 elements (i.e. slices).
      | 
      | Use BRAM for Twiddle Coefficients (twiddle_bram): Check this checkbox to store twiddle
      | coefficients in BRAM.  If unchecked, the twiddle coefficients will be sored in distributed
      | memory (i.e. slices).
      | 
      | Twiddle Coefficient Bitwidth (n_bits_w): Specifies the width of the real/imaginary
      | components of the twiddle coefficients.  Assumed equal for both components.
      | 
      | Multiplier Latency (mult_latency): Latency to use for the underlying real multipliers.
      | 
      | Adder Latency (add_latency): Latency to use for the underlying real adders.
      | </pre>
  a_out : Outport  OutDataType=sfix(16)  OutScaling=2^0
  b_out : Outport  Port=2  OutDataType=sfix(16)  OutScaling=2^0
  sync_out : Outport  Port=3  OutDataType=sfix(16)  OutScaling=2^0
  wires:
  a_in/1 -> r2_dit_stage_1/1(a_in)
  b_in/1 -> r2_dit_stage_1/2(b_in)
  sync_in/1 -> r2_dit_stage_1/3(sync_in)
  r2_dit_stage_1/1(a_out) -> r2_dit_stage_2/1(a_in)
  r2_dit_stage_1/2(b_out) -> r2_dit_stage_2/2(b_in)
  r2_dit_stage_1/3(sync_out) -> r2_dit_stage_2/3(sync_in)
  r2_dit_stage_2/1(a_out) -> biplex_commutator/1(AloAhi)
  r2_dit_stage_2/2(b_out) -> biplex_commutator/2(BloBhi)
  r2_dit_stage_2/3(sync_out) -> biplex_commutator/3(sync_in)
  biplex_commutator/1(AloBlo) -> biplex_bitrev/1(a_in)
  biplex_commutator/2(AhiBhi) -> biplex_bitrev/2(b_in)
  biplex_commutator/3(sync_out) -> biplex_bitrev/3(sync_in)
  biplex_bitrev/1(a_out) -> a_out/1
  biplex_bitrev/2(b_out) -> b_out/1
  biplex_bitrev/3(sync_out) -> sync_out/1

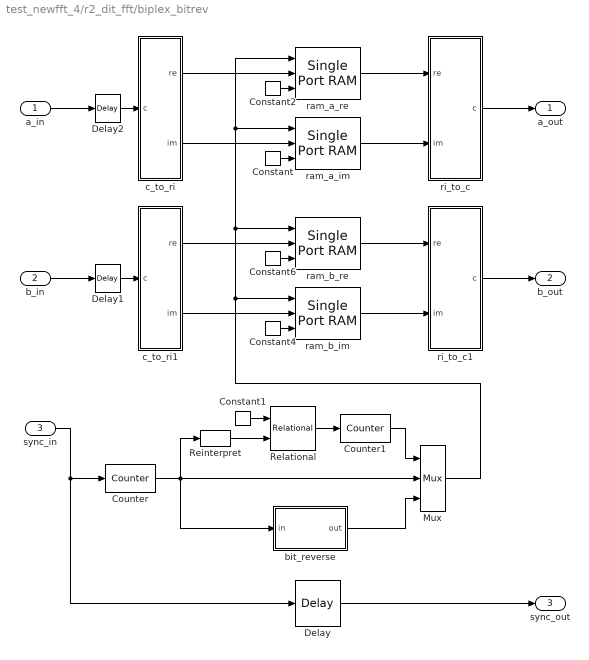
== system test_newfft_4/r2_dit_fft/biplex_bitrev ==
  a_in : Inport  OutDataType=sfix(16)  OutScaling=2^0
  b_in : Inport  Port=2  OutDataType=sfix(16)  OutScaling=2^0
  sync_in : Inport  Port=3  OutDataType=sfix(16)  OutScaling=2^0
  Constant{,2,4,6} (4 alike) : xbsIndex_r4/Constant  arith_type=Boolean  const=1  n_bits=1  bin_pt=0  explicit_period=on  period=1  equ=P=C  opselect=C  inp2=PCIN>>17  opr=+  inp1=P  carry=CIN  dbl_ovrd=off  block_type=constant
  Constant1 : xbsIndex_r4/Constant  arith_type=Signed (2's comp)  const=-1  n_bits=1  bin_pt=0  explicit_period=on  period=1  equ=P=C  opselect=C  inp2=PCIN>>17  opr=+  inp1=P  carry=CIN  dbl_ovrd=off  block_type=constant
  Counter : xbsIndex_r4/Counter  cnt_type=Free Running  cnt_to=Inf  operation=Up  start_count=0  cnt_by_val=1  arith_type=Unsigned  n_bits=1  bin_pt=0  load_pin=off  rst=on  en=off  explicit_period=off  period=1  dbl_ovrd=off  use_behavioral_HDL=off  use_rpm=on  implementation=Fabric  block_type=counter
      settings: xl_area=[0, 0, 0, 0, 0, 0, 0]
  Counter1 : xbsIndex_r4/Counter  cnt_type=Free Running  cnt_to=Inf  operation=Up  start_count=0  cnt_by_val=1  arith_type=Unsigned  n_bits=1  bin_pt=0  load_pin=off  rst=off  en=on  explicit_period=off  period=1  dbl_ovrd=off  use_behavioral_HDL=off  use_rpm=on  implementation=Fabric  block_type=counter
      settings: xl_area=[0, 0, 0, 0, 0, 0, 0]
  Delay : xbsIndex_r4/Delay  en=off  latency=4  dbl_ovrd=off  reg_retiming=off  block_type=delay
      settings: xl_area=[0, 0, 0, 0, 0, 0, 0]
  Delay1 : xbsIndex_r4/Delay  en=off  latency=1  dbl_ovrd=off  reg_retiming=off  block_type=delay
      settings: xl_area=[0, 0, 0, 0, 0, 0, 0]
  Delay2 : xbsIndex_r4/Delay  en=off  latency=1  dbl_ovrd=off  reg_retiming=off  block_type=delay
      settings: xl_area=[0, 0, 0, 0, 0, 0, 0]
  Mux : xbsIndex_r4/Mux  inputs=2  en=off  latency=1  precision=Full  arith_type="Signed  (2's comp)"  n_bits=8  bin_pt=2  quantization=Truncate  overflow=Wrap  dbl_ovrd=off  block_type=mux
      settings: xl_area=[0, 0, 0, 0, 0, 0, 0]
  Reinterpret : xbsIndex_r4/Reinterpret  force_arith_type=on  arith_type="Signed  (2's comp)"  force_bin_pt=off  bin_pt=0  block_type=reinterpret
      settings: infoedit="Changes signal type without altering the binary representation.   You can changed the signal between signed and unsigned, and relocate the binary point.<P><P>Hardware notes: In hardware this block costs nothing.<P><P>Example:  Suppose the input is 6 bits wide, signed, with 2 fractional bits, and the output is forced to unsigned with 0 fractional bits.  Then an input of -2.0 (1110.00 in binary 2's complement) becomes an output of 56 (111000 in binary)."  block_version=10.1.3
  Relational : xbsIndex_r4/Relational  mode=a=b  en=off  latency=1  dbl_ovrd=off  block_type=relational
      settings: xl_area=[0, 0, 0, 0, 0, 0, 0]  block_version=10.1.3
  bit_reverse : Subsystem  mask(Bit Reversal){n_bits=1}
      mask prompts: n_bits "Number of Bits"
      mask help: Reverses the bit order of the input. Input must be unsigned with binary point at position 0. Costs nothing in hardware.
      settings: AttributesFormatString=1 bits
      mask Help:
      | <pre>
      | Description::
      | 
      | Reverses the bit order of the input.
      | 
      | Input must be unsigned with binary point at position 0.
      | 
      | Costs nothing in hardware.
      | 
      | Mask Parameters::
      | 
      | Number of Bits (n_bits): Specifies the width of the input.
      | </pre>
  c_to_ri : Subsystem  mask(Complex to Real-Imag){n_bits=10, bin_pt=0}
      mask prompts: n_bits "Bit Width"; bin_pt "Binary Point"
      mask help: Outputs real and imaginary components of a complex input.
      settings: AttributesFormatString=10_0 r/i
      mask Help:
      | <pre>
      | Description::
      | 
      | Outputs real and imaginary components of a complex input.
      | Useful for simplifying interconnects.
      | See also: Real-Imag to Complex (ri_to_c)
      | 
      | Mask Parameters::
      | 
      | Bit Width (n_bits): Specifies the width of the real/imaginary components.
      | Assumed equal for both components.
      | 
      | Binary Point (bin_pt): Specifies the binary point location in the real/imaginary components.
      | Assumed equal for both components.
      | </pre>
  c_to_ri1 : Subsystem  mask(Complex to Real-Imag){n_bits=10, bin_pt=0}
      mask prompts: n_bits "Bit Width"; bin_pt "Binary Point"
      mask help: Outputs real and imaginary components of a complex input.
      settings: AttributesFormatString=10_0 r/i
      mask Help:
      | <pre>
      | Description::
      | 
      | Outputs real and imaginary components of a complex input.
      | Useful for simplifying interconnects.
      | See also: Real-Imag to Complex (ri_to_c)
      | 
      | Mask Parameters::
      | 
      | Bit Width (n_bits): Specifies the width of the real/imaginary components.
      | Assumed equal for both components.
      | 
      | Binary Point (bin_pt): Specifies the binary point location in the real/imaginary components.
      | Assumed equal for both components.
      | </pre>
  ram_a_im : xbsIndex_r4/Single Port RAM  depth=2  initVector=0  distributed_mem=Block RAM  write_mode=Read Before Write  rst=off  init_reg=0  en=off  latency=1  dbl_ovrd=off  optimize=Area  use_rpm=off  block_type=spram
      settings: xl_area=[0, 0, 0, 0, 0, 0, 0]  block_version=10.1.3
  ram_a_re : xbsIndex_r4/Single Port RAM  depth=2  initVector=0  distributed_mem=Block RAM  write_mode=Read Before Write  rst=off  init_reg=0  en=off  latency=1  dbl_ovrd=off  optimize=Area  use_rpm=off  block_type=spram
      settings: xl_area=[0, 0, 0, 0, 0, 0, 0]  block_version=10.1.3
  ram_b_im : xbsIndex_r4/Single Port RAM  depth=2  initVector=0  distributed_mem=Block RAM  write_mode=Read Before Write  rst=off  init_reg=0  en=off  latency=1  dbl_ovrd=off  optimize=Area  use_rpm=off  block_type=spram
      settings: xl_area=[0, 0, 0, 0, 0, 0, 0]  block_version=10.1.3
  ram_b_re : xbsIndex_r4/Single Port RAM  depth=2  initVector=0  distributed_mem=Block RAM  write_mode=Read Before Write  rst=off  init_reg=0  en=off  latency=1  dbl_ovrd=off  optimize=Area  use_rpm=off  block_type=spram
      settings: xl_area=[0, 0, 0, 0, 0, 0, 0]  block_version=10.1.3
  ri_to_c : Subsystem
      mask Type: Real-Imag to Complex
      mask Description: Concatenates real and imaginary inputs into a complex output.
      mask Help:
      | <pre>
      | Description::
      | 
      | Concatenates a real and imaginary input into a complex output.
      | Useful for simplifying interconnects.
      | See also: Complex to Real-Imag (c_to_ri)
      | 
      | Mask Parameters::
      | 
      | (N/A)
      | </pre>
  ri_to_c1 : Subsystem
      mask Type: Real-Imag to Complex
      mask Description: Concatenates real and imaginary inputs into a complex output.
      mask Help:
      | <pre>
      | Description::
      | 
      | Concatenates a real and imaginary input into a complex output.
      | Useful for simplifying interconnects.
      | See also: Complex to Real-Imag (c_to_ri)
      | 
      | Mask Parameters::
      | 
      | (N/A)
      | </pre>
  a_out : Outport  OutDataType=sfix(16)  OutScaling=2^0
  b_out : Outport  Port=2  OutDataType=sfix(16)  OutScaling=2^0
  sync_out : Outport  Port=3  OutDataType=sfix(16)  OutScaling=2^0
  wires:
  Reinterpret/1 -> Relational/2
  Relational/1 -> Counter1/1
  Constant1/1 -> Relational/1
  Counter1/1 -> Mux/1
  Counter/1 -> Reinterpret/1, Mux/2, bit_reverse/1(in)
  Constant6/1 -> ram_b_re/3
  Constant4/1 -> ram_b_im/3
  Constant2/1 -> ram_a_re/3
  Constant/1 -> ram_a_im/3
  Delay/1 -> sync_out/1
  Mux/1 -> ram_b_im/1, ram_b_re/1, ram_a_im/1, ram_a_re/1
  bit_reverse/1(out) -> Mux/3
  b_in/1 -> Delay1/1
  a_in/1 -> Delay2/1
  c_to_ri1/2(im) -> ram_b_im/2
  c_to_ri1/1(re) -> ram_b_re/2
  c_to_ri/2(im) -> ram_a_im/2
  c_to_ri/1(re) -> ram_a_re/2
  ri_to_c1/1(c) -> b_out/1
  ri_to_c/1(c) -> a_out/1
  ram_b_im/1 -> ri_to_c1/2(im)
  ram_b_re/1 -> ri_to_c1/1(re)
  ram_a_im/1 -> ri_to_c/2(im)
  ram_a_re/1 -> ri_to_c/1(re)
  sync_in/1 -> Delay/1, Counter/1
  Delay1/1 -> c_to_ri1/1(c)
  Delay2/1 -> c_to_ri/1(c)
